simulink model "PathFollowComp"  (R2015a)
settings: Solver=ode3  StartTime=0.0  StopTime=400  FixedStep=0.01  RelTol=1e-3
values from neighbouring files (symbols this model uses):
  K_eta = 1    [CD.m]    (also in PathFollowCompScript.m = 0.21)
  lambda_0 = atan2(lambda_vec_0(2),lambda_vec_0(1))    [CD.m]    (also in PathFollowCompScript.m)
  rangethresh = 50    [PathFollowCompScript.m]
undefined symbols (not defined in the file): Initial_Heading, Initial_Position, Initial_Position_O
libraries: simulink x13, aerolibtransform2 x4
(part 1 of 2)
settings Model: Creator=marinho  LastModifiedBy=marinho

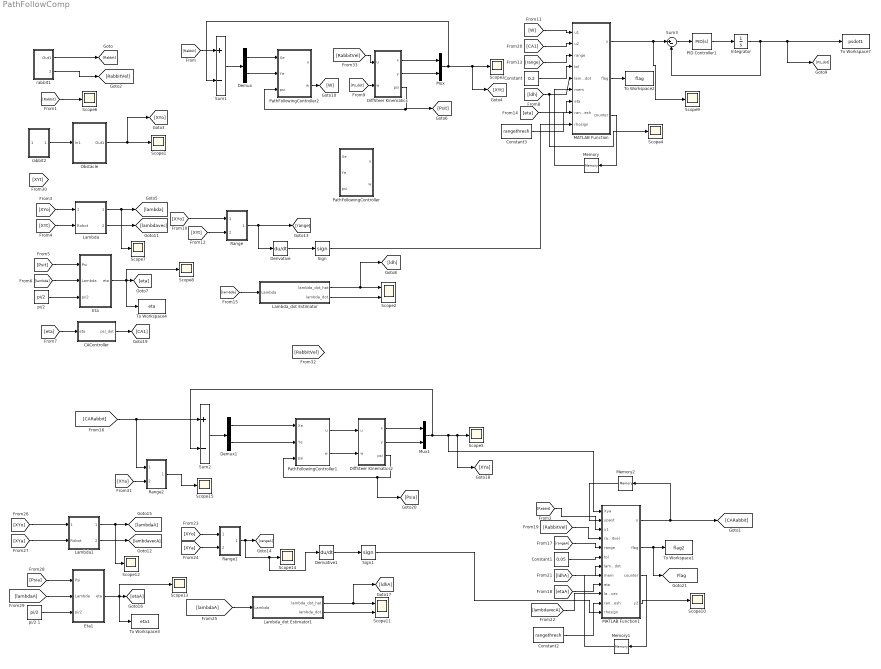
== system PathFollowComp ==
  CAController : Subsystem
  Constant : Constant  Value=0.2
  Constant1 : Constant  Value=0.05
  Constant2 : Constant  Value=rangethresh
  Constant3 : Constant  Value=rangethresh
  Demux : Demux  Outputs=2
  Demux1 : Demux  Outputs=2
  Derivative : Derivative
  Derivative1 : Derivative
  DiffSteer Kinematics : Subsystem  AncestorBlock=DiffSteer_model/DiffSteer Kinematics  mask{x0=[Initial_Position Initial_Heading], a=0.2, umax=32, wmax=5, dumax=inf, dwmax=inf}
      mask prompts: x0 "Initial pose [x, y, psi]"; a "Distance from traction wheels axis center to the point of interest [m]"; umax "Maximum linear velocity [m/s]"; wmax "Maximum angular velocity [rad/s]"; dumax "Maximum linear acceleration [m/s^2]"; dwmax "Maximum angular acceleration [rad/s^2]"
      mask help: Kinematics of the differential steered vehicle
      mask Help:
      | Kinematics of the differential steered vehicle (unicycle-like).
      | 
      | A differential steered (or differential wheeled) robot has two separately driven wheels placed on either side of its structure. Its orientation is changed by varying the relative velocities of its wheels.
      | In this model, robot position [x,y] is the position of the point of interest, which is located on a distance "a" from the center of the line that connects both traction wheels. If a = 0, this model is equal to the unicycle.
      | 
      | <b>Parameters:</b>
      | 
      | Initial pose: Vehicle initial position and orientation on absolute reference frame [x_0, y_0, psi_0]
      | Distance between traction wheels axis and point of interest (1x1): a [m]
      | Maximum Linear velocity (1x1):  Vehicle speed limit [m/s] (umax)
      | Maximum Angular velocity (1x1):  Vehicle turning velocity limit [rad/s] (wmax)
      | Maximum linear acceleration (1x1): Vehicle linear acceleration limit [m/s2] (dumax)
      | Maximum angular acceleration (1x1): Vehicle angular acceleration limit [rad/s2] (dwmax)
      | 
      | 
      | <b>Inputs:</b>
      | 
      | u (1x1): reference for linear velocity [m/s]
      | w (1x1): reference for angular velocity [rad/s]
      | 
      | <b>Outputs:</b>
      | 
      | x (1x1): x-coordinate in world frame [m]
      | y (1x1): y-coordinate in world frame [m]
      | psi (1x1): heading angle in world frame [rad]
      | 
      | <b>Notes:</b>
      | 
      | 1. If a = 0, this model is equal to the unicycle.
      | 
      | 2. This model does not take into account the robot dynamics. It considers that the actual robot velocity is exactly equal to the reference velocity (if it is bellow its limit).
      | 
      | For more information on the robot kinematics and dynamics, please refer to:
      | 
      | [1] MARTINS, F.N., CARELLI, R., SARCINELLI-FILHO, M. and BASTOS-FILHO, T.F.
      | Dynamic Modeling and Adaptive Dynamic Compensation for Unicycle-Like
      | Mobile Robots. 14th International Conference on Advanced Robotics -
      | ICAR 2009, Germany, June, 22-26, 2009.
      | 
      | [2] MARTINS, F.N., CELESTE, W.C., CARELLI, R., SARCINELLI-FILHO, M. and
      | BASTOS-FILHO, T.F. An Adaptive Dynamic Controller for Autonomous Mobile Robot
      | Trajectory Tracking. Control Engineering Practice, v. 16, p. 1354–1363, 2008.
      | doi: 10.1016/j.conengprac.2008.03.004
  DiffSteer Kinematics2 : Subsystem  AncestorBlock=DiffSteer_model/DiffSteer Kinematics  mask{x0=[Initial_Position Initial_Heading], a=0.2, umax=32, wmax=5, dumax=inf, dwmax=inf}
      mask prompts: x0 "Initial pose [x, y, psi]"; a "Distance from traction wheels axis center to the point of interest [m]"; umax "Maximum linear velocity [m/s]"; wmax "Maximum angular velocity [rad/s]"; dumax "Maximum linear acceleration [m/s^2]"; dwmax "Maximum angular acceleration [rad/s^2]"
      mask help: Kinematics of the differential steered vehicle
      mask Help:
      | Kinematics of the differential steered vehicle (unicycle-like).
      | 
      | A differential steered (or differential wheeled) robot has two separately driven wheels placed on either side of its structure. Its orientation is changed by varying the relative velocities of its wheels.
      | In this model, robot position [x,y] is the position of the point of interest, which is located on a distance "a" from the center of the line that connects both traction wheels. If a = 0, this model is equal to the unicycle.
      | 
      | <b>Parameters:</b>
      | 
      | Initial pose: Vehicle initial position and orientation on absolute reference frame [x_0, y_0, psi_0]
      | Distance between traction wheels axis and point of interest (1x1): a [m]
      | Maximum Linear velocity (1x1):  Vehicle speed limit [m/s] (umax)
      | Maximum Angular velocity (1x1):  Vehicle turning velocity limit [rad/s] (wmax)
      | Maximum linear acceleration (1x1): Vehicle linear acceleration limit [m/s2] (dumax)
      | Maximum angular acceleration (1x1): Vehicle angular acceleration limit [rad/s2] (dwmax)
      | 
      | 
      | <b>Inputs:</b>
      | 
      | u (1x1): reference for linear velocity [m/s]
      | w (1x1): reference for angular velocity [rad/s]
      | 
      | <b>Outputs:</b>
      | 
      | x (1x1): x-coordinate in world frame [m]
      | y (1x1): y-coordinate in world frame [m]
      | psi (1x1): heading angle in world frame [rad]
      | 
      | <b>Notes:</b>
      | 
      | 1. If a = 0, this model is equal to the unicycle.
      | 
      | 2. This model does not take into account the robot dynamics. It considers that the actual robot velocity is exactly equal to the reference velocity (if it is bellow its limit).
      | 
      | For more information on the robot kinematics and dynamics, please refer to:
      | 
      | [1] MARTINS, F.N., CARELLI, R., SARCINELLI-FILHO, M. and BASTOS-FILHO, T.F.
      | Dynamic Modeling and Adaptive Dynamic Compensation for Unicycle-Like
      | Mobile Robots. 14th International Conference on Advanced Robotics -
      | ICAR 2009, Germany, June, 22-26, 2009.
      | 
      | [2] MARTINS, F.N., CELESTE, W.C., CARELLI, R., SARCINELLI-FILHO, M. and
      | BASTOS-FILHO, T.F. An Adaptive Dynamic Controller for Autonomous Mobile Robot
      | Trajectory Tracking. Control Engineering Practice, v. 16, p. 1354–1363, 2008.
      | doi: 10.1016/j.conengprac.2008.03.004
  Eta : Subsystem
  Eta1 : Subsystem
  Integrator : Integrator  UpperSaturationLimit=0.5  LowerSaturationLimit=-0.5
  Lambda : Subsystem
  Lambda1 : Subsystem
  Lambda_dot Estimator : Subsystem
  Lambda_dot Estimator1 : Subsystem
  MATLAB Function : MATLAB Function  TreatAsAtomicUnit=on
  MATLAB Function1 : MATLAB Function  TreatAsAtomicUnit=on
  Memory : Memory
  Memory1 : Memory
  Memory2 : Memory  X0=[0 0]'
  Mux : Mux  Inputs=2
  Mux1 : Mux  Inputs=2
  Obstacle : Subsystem
  PID Controller1 : simulink/Continuous/PID Controller  Controller=PID  TimeDomain=Continuous-time  SampleTime=-1  IntegratorMethod=Forward Euler  FilterMethod=Forward Euler  Form=Parallel  UseFilter=on  ControllerParametersSource=internal  P=1  I=0  D=0.05  N=100  InitialConditionSource=internal  InitialConditionForIntegrator=0  InitialConditionForFilter=0  ExternalReset=none  LimitOutput=off  UpperSaturationLimit=0.1  LowerSaturationLimit=-0.1  LinearizeAsGain=on  AntiWindupMode=none  Kb=1  TrackingMode=off  Kt=1  PParamMin=[]  PParamMax=[]  IParamMin=[]  IParamMax=[]  DParamMin=[]  DParamMax=[]  NParamMin=[]  NParamMax=[]  KbParamMin=[]  KbParamMax=[]  KtParamMin=[]  KtParamMax=[]  POutMin=[]  POutMax=[]  IOutMin=[]  IOutMax=[]  DOutMin=[]  DOutMax=[]  NOutMin=[]  NOutMax=[]  KbOutMin=[]  KbOutMax=[]  KtOutMin=[]  KtOutMax=[]  IntegratorOutMin=[]  IntegratorOutMax=[]  FilterOutMin=[]  FilterOutMax=[]  SumOutMin=[]  SumOutMax=[]  SumI1OutMin=[]  SumI1OutMax=[]  SumI2OutMin=[]  SumI2OutMax=[]  SumI3OutMin=[]  SumI3OutMax=[]  SumDOutMin=[]  SumDOutMax=[]  SaturationOutMin=[]  SaturationOutMax=[]  IntegratorContinuousStateAttributes=''  IntegratorStateMustResolveToSignalObject=off  IntegratorRTWStateStorageClass=Auto  FilterContinuousStateAttributes=''  FilterStateMustResolveToSignalObject=off  FilterRTWStateStorageClass=Auto  DifferentiatorICPrevScaledInput=0  DifferentiatorOutMin=[]  DifferentiatorOutMax=[]
  PathFollowingController : Subsystem
  PathFollowingController1 : Subsystem
  PathFollowingController2 : Subsystem
  Range : Subsystem
  Range1 : Subsystem
  Range2 : Subsystem
  Scope{1,3..10,12..15} (13 alike) : Scope
      Scope1 settings: YMin=-250  YMax=25  SaveName=Obstacle
      Scope10 settings: SaveName=NewRabbit
      Scope12 settings: SaveName=Cdc5  DataFormat=Structure
      Scope13 settings: SaveName=Cdc6  DataFormat=Structure
      Scope14 settings: YMin=50  YMax=425  SaveName=Range
      Scope15 settings: YMin=85  YMax=160  SaveName=NewRabbit1
      Scope3 settings: SaveName=Cdc  DataFormat=Structure
      Scope4 settings: SaveName=Cdc1  DataFormat=Structure
      Scope5 settings: SaveName=AlphaBased  DataFormat=Structure
      Scope6 settings: SaveName=Rabbit
      Scope7 settings: SaveName=Cdc2  DataFormat=Structure
      Scope8 settings: SaveName=Cdc3  DataFormat=Structure
      Scope9 settings: SaveName=Cdc4  DataFormat=Structure
  Scope11 : Scope  NumInputPorts=2
      settings: YMin=-5~-5  YMax=5~5
  Scope2 : Scope  NumInputPorts=2
      settings: YMin=-1~-5  YMax=12~70  SaveName=ScopeData10
  Sign : Signum
  Sign1 : Signum
  Sum1 : Sum  Inputs=+-
  Sum2 : Sum  Inputs=+-
  Sum3 : Sum  Inputs=|+-
  To Workspace1 : ToWorkspace  VariableName=flag2  SampleTime=-1
  To Workspace2 : ToWorkspace  VariableName=flag  SampleTime=-1
  To Workspace3 : ToWorkspace  VariableName=eta1  SampleTime=-1
  To Workspace4 : ToWorkspace  VariableName=eta  SampleTime=-1
  To Workspace7 : ToWorkspace  VariableName=psdot1  SampleTime=-1
  "pi/2 " : Constant  Value=pi/2  VectorParams1D=off  SampleTime=-1
  pi/2 1 : Constant  Value=pi/2  VectorParams1D=off  SampleTime=-1
  rabbit1 : Subsystem
  rabbit2 : Subsystem
  tag scope: Flag=global
  wires:
  DiffSteer Kinematics/1(x) -> Mux/1
  DiffSteer Kinematics/2(y) -> Mux/2
  Sum1/1 -> Demux/1
  Demux/2 -> PathFollowingController2/2(Ye)
  Demux/1 -> PathFollowingController2/1(Xe)
  Mux/1 -> Sum1/2, [XYt], Scope3/1
  DiffSteer Kinematics/3(psi) -> PathFollowingController2/3(psi), [Psit]
  DiffSteer Kinematics2/1(x) -> Mux1/1
  DiffSteer Kinematics2/2(y) -> Mux1/2
  Sum2/1 -> Demux1/1
  Demux1/2 -> PathFollowingController1/2(Ye)
  Demux1/1 -> PathFollowingController1/1(Xe)
  Mux1/1 -> Sum2/2, MATLAB Function1/1(Xya), [XYa], Scope5/1
  PathFollowingController1/2(w) -> DiffSteer Kinematics2/2(w)
  DiffSteer Kinematics2/3(psi) -> [Psia], PathFollowingController1/3(psi)
  rabbit1/1(Out1) -> [Rabbit]
  [Rabbit] -> Sum1/1
  [Rabbit] -> Scope6/1
  [XYo] -> Lambda/1(Object)
  [XYt] -> Lambda/2(Robot)
  Lambda/1(Lambda) -> Scope7/1, [lambda]
  Eta/1(eta) -> To Workspace4/1, Scope8/1, [eta]
  [Psit] -> Eta/1(Psi)
  [lambda] -> Eta/2(Lambda)
  "pi/2 "/1 -> Eta/3(pi/2)
  [eta] -> CAController/1(eta)
  CAController/1(psi_dot) -> [CA1]
  [W] -> MATLAB Function/1(u1)
  MATLAB Function/2(flag) -> To Workspace2/1
  [range] -> MATLAB Function/3(range)
  MATLAB Function/3(counter) -> Memory/1
  Memory/1 -> MATLAB Function/6(mem)
  Constant/1 -> MATLAB Function/4(tol)
  [eta] -> MATLAB Function/7(eta)
  [ldh] -> Scope4/1, MATLAB Function/5(lambda_dot)
  Sum3/1 -> PID Controller1/1
  PID Controller1/1 -> Integrator/1
  MATLAB Function/1(y) -> Scope9/1, Sum3/1
  Integrator/1 -> [Ps_dot], To Workspace7/1, Sum3/2
  [CA1] -> MATLAB Function/2(u2)
  PathFollowingController2/2(w) -> [W]
  [Ps_dot] -> DiffSteer Kinematics/2(w)
  [XYo] -> Range/1(In1)
  [XYt] -> Range/2(In2)
  Range/1(Out1) -> Derivative/1, [range]
  [lambda] -> Lambda_dot Estimator/1(Lambda)
  Lambda_dot Estimator/1(lambda_dot_hat) -> [ldh], Scope2/1
  Lambda_dot Estimator/2(lambda_dot) -> Scope2/2
  [Rabbit] -> MATLAB Function1/3(u1)
  [rangeA] -> MATLAB Function1/5(range)
  MATLAB Function1/3(counter) -> Memory1/1
  Memory1/1 -> MATLAB Function1/8(mem)
  Constant1/1 -> MATLAB Function1/6(tol)
  [etaA] -> MATLAB Function1/9(eta)
  [ldhA] -> MATLAB Function1/7(lambda_dot)
  MATLAB Function1/1(y) -> Memory2/1, [CARabbit]
  [CARabbit] -> Range2/1(In1), Sum2/1
  rabbit1/2(Velocity) -> [RabbitVel]
  [RabbitVel] -> MATLAB Function1/4(rabbitvel)
  Lambda/2(LambdaVec) -> [lambdavec]
  [lambdavecA] -> MATLAB Function1/10(lambdavec)
  MATLAB Function1/4(y2) -> Scope10/1
  Memory2/1 -> MATLAB Function1/2(ypast)
  Constant2/1 -> MATLAB Function1/11(rangethresh)
  Constant3/1 -> MATLAB Function/8(rangethresh)
  [XYo] -> Lambda1/1(Object)
  [XYa] -> Lambda1/2(Robot)
  Lambda1/1(Lambda) -> Scope12/1, [lambdaA]
  Eta1/1(eta) -> To Workspace3/1, Scope13/1, [etaA]
  [Psia] -> Eta1/1(Psi)
  [lambdaA] -> Eta1/2(Lambda)
  pi/2 1/1 -> Eta1/3(pi/2)
  [XYo] -> Range1/1(In1)
  [XYa] -> Range1/2(In2)
  Range1/1(Out1) -> Derivative1/1, Scope14/1, [rangeA]
  [lambdaA] -> Lambda_dot Estimator1/1(Lambda)
  Lambda_dot Estimator1/1(lambda_dot_hat) -> [ldhA], Scope11/1
  Lambda_dot Estimator1/2(lambda_dot) -> Scope11/2
  Lambda1/2(LambdaVec) -> [lambdavecA]
  Obstacle/1(Out1) -> [XYo], Scope1/1
  Derivative/1 -> Sign/1
  Sign/1 -> MATLAB Function/9(rhosign)
  Derivative1/1 -> Sign1/1
  Sign1/1 -> MATLAB Function1/12(rhosign)
  [XYa] -> Range2/2(In2)
  Range2/1(Out1) -> Scope15/1
  MATLAB Function1/2(flag) -> [Flag], To Workspace1/1
  rabbit2/1(Out1) -> Obstacle/1(In1)
  [RabbitVel] -> DiffSteer Kinematics/1(u)
  PathFollowingController1/1(u) -> DiffSteer Kinematics2/1(u)

== system PathFollowComp/CAController ==
  eta : Inport
  Gain : Gain  Gain=-K_eta
  psi_dot : Outport
  wires:
  Gain/1 -> psi_dot/1
  eta/1 -> Gain/1

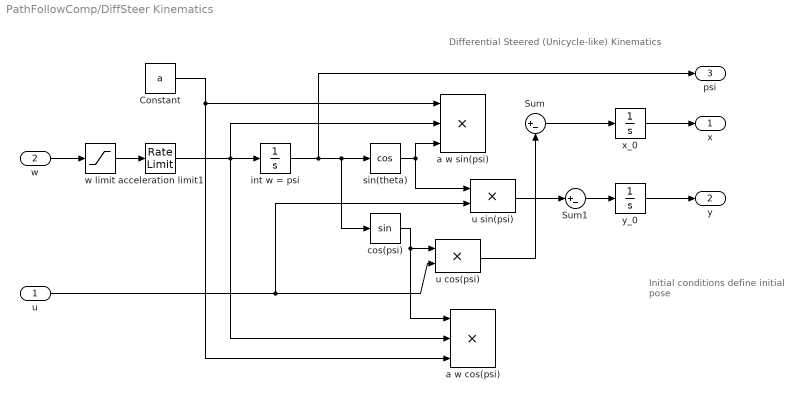
== system PathFollowComp/DiffSteer Kinematics ==
  note: Initial conditions define
      | initial pose
  note: Differential Steered (Unicycle-like) Kinematics
  u : Inport
  w : Inport  Port=2
  Constant : Constant  Value=a
  Sum : Sum  Inputs=|+-  SaturateOnIntegerOverflow=on
  Sum1 : Sum  Inputs=|+-  SaturateOnIntegerOverflow=on
  a w cos(psi) : Product  Inputs=3  SaturateOnIntegerOverflow=on  OutDataTypeStr=Inherit: Same as first input
  a w sin(psi) : Product  Inputs=3  SaturateOnIntegerOverflow=on  OutDataTypeStr=Inherit: Same as first input
  acceleration limit1 : RateLimiter  RisingSlewLimit=dwmax  FallingSlewLimit=-dwmax  SampleTimeMode=inherited
  cos(psi) : Trigonometry
  int w = psi : Integrator  InitialCondition=x0(3)
  sin(theta) : Trigonometry  Operator=cos
  u cos(psi) : Product  SaturateOnIntegerOverflow=on  OutDataTypeStr=Inherit: Same as first input
  u sin(psi) : Product  SaturateOnIntegerOverflow=on  OutDataTypeStr=Inherit: Same as first input
  w limit : Saturate  UpperLimit=wmax  LowerLimit=-wmax
  x_0 : Integrator  InitialCondition=x0(1)
  y_0 : Integrator  InitialCondition=x0(2)
  x : Outport
  y : Outport  Port=2
  psi : Outport  Port=3
  wires:
  w limit/1 -> acceleration limit1/1
  w/1 -> w limit/1
  u cos(psi)/1 -> Sum/2
  u sin(psi)/1 -> Sum1/1
  cos(psi)/1 -> u cos(psi)/1, a w cos(psi)/1
  acceleration limit1/1 -> a w sin(psi)/2, int w = psi/1, a w cos(psi)/2
  Constant/1 -> a w sin(psi)/1, a w cos(psi)/3
  x_0/1 -> x/1
  Sum/1 -> x_0/1
  sin(theta)/1 -> a w sin(psi)/3, u sin(psi)/1
  int w = psi/1 -> psi/1, sin(theta)/1, cos(psi)/1
  u/1 -> u sin(psi)/2, u cos(psi)/2
  Sum1/1 -> y_0/1
  y_0/1 -> y/1

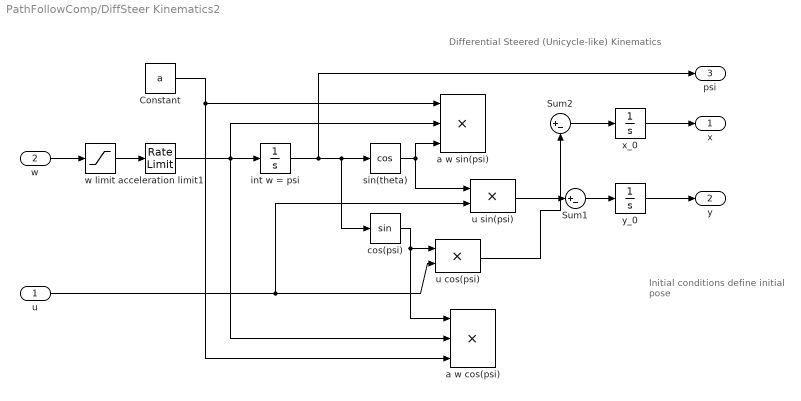
== system PathFollowComp/DiffSteer Kinematics2 ==
  note: Initial conditions define
      | initial pose
  note: Differential Steered (Unicycle-like) Kinematics
  u : Inport
  w : Inport  Port=2
  Constant : Constant  Value=a
  Sum1 : Sum  Inputs=|+-  SaturateOnIntegerOverflow=on
  Sum2 : Sum  Inputs=|+-  SaturateOnIntegerOverflow=on
  a w cos(psi) : Product  Inputs=3  SaturateOnIntegerOverflow=on  OutDataTypeStr=Inherit: Same as first input
  a w sin(psi) : Product  Inputs=3  SaturateOnIntegerOverflow=on  OutDataTypeStr=Inherit: Same as first input
  acceleration limit1 : RateLimiter  RisingSlewLimit=dwmax  FallingSlewLimit=-dwmax  SampleTimeMode=inherited
  cos(psi) : Trigonometry
  int w = psi : Integrator  InitialCondition=x0(3)
  sin(theta) : Trigonometry  Operator=cos
  u cos(psi) : Product  SaturateOnIntegerOverflow=on  OutDataTypeStr=Inherit: Same as first input
  u sin(psi) : Product  SaturateOnIntegerOverflow=on  OutDataTypeStr=Inherit: Same as first input
  w limit : Saturate  UpperLimit=wmax  LowerLimit=-wmax
  x_0 : Integrator  InitialCondition=x0(1)
  y_0 : Integrator  InitialCondition=x0(2)
  x : Outport
  y : Outport  Port=2
  psi : Outport  Port=3
  wires:
  w limit/1 -> acceleration limit1/1
  w/1 -> w limit/1
  u sin(psi)/1 -> Sum1/1
  cos(psi)/1 -> u cos(psi)/1, a w cos(psi)/1
  acceleration limit1/1 -> a w sin(psi)/2, int w = psi/1, a w cos(psi)/2
  Constant/1 -> a w sin(psi)/1, a w cos(psi)/3
  x_0/1 -> x/1
  u cos(psi)/1 -> Sum2/2
  sin(theta)/1 -> a w sin(psi)/3, u sin(psi)/1
  int w = psi/1 -> psi/1, sin(theta)/1, cos(psi)/1
  u/1 -> u sin(psi)/2, u cos(psi)/2
  Sum1/1 -> y_0/1
  y_0/1 -> y/1
  Sum2/1 -> x_0/1

== system PathFollowComp/Eta ==
  Psi : Inport
  Lambda : Inport  Port=2
  pi/2 : Inport  Port=3
  Gain5 : Gain
  Sum2 : Sum  Inputs=+-
  Sum3 : Sum  Inputs=+-
  wrap1 : MATLAB Function  TreatAsAtomicUnit=on
  eta : Outport
  wires:
  wrap1/1(y) -> eta/1
  Psi/1 -> Gain5/1
  Lambda/1 -> Sum3/1
  Sum3/1 -> Sum2/2
  pi/2/1 -> Sum3/2
  Sum2/1 -> wrap1/1(u)
  Gain5/1 -> Sum2/1

== system PathFollowComp/Eta1 ==
  Psi : Inport
  Lambda : Inport  Port=2
  pi/2 : Inport  Port=3
  Gain5 : Gain
  Sum2 : Sum  Inputs=+-
  Sum3 : Sum  Inputs=+-
  wrap1 : MATLAB Function  TreatAsAtomicUnit=on
  eta : Outport
  wires:
  wrap1/1(y) -> eta/1
  Psi/1 -> Gain5/1
  Lambda/1 -> Sum3/1
  Sum3/1 -> Sum2/2
  pi/2/1 -> Sum3/2
  Sum2/1 -> wrap1/1(u)
  Gain5/1 -> Sum2/1

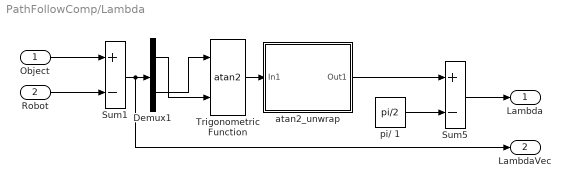
== system PathFollowComp/Lambda ==
  Object : Inport
  Robot : Inport  Port=2
  Demux1 : Demux  Outputs=2
  Sum1 : Sum  Inputs=+-
  Sum5 : Sum  Inputs=+-
  Trigonometric Function : Trigonometry  Operator=atan2
  atan2_unwrap : Subsystem
  pi/ 1 : Constant  Value=pi/2  VectorParams1D=off  SampleTime=-1
  Lambda : Outport
  LambdaVec : Outport  Port=2
  wires:
  Trigonometric Function/1 -> atan2_unwrap/1(In1)
  Demux1/2 -> Trigonometric Function/1
  pi/ 1/1 -> Sum5/2
  Sum5/1 -> Lambda/1
  atan2_unwrap/1(Out1) -> Sum5/1
  Sum1/1 -> LambdaVec/1, Demux1/1
  Demux1/1 -> Trigonometric Function/2
  Object/1 -> Sum1/1
  Robot/1 -> Sum1/2

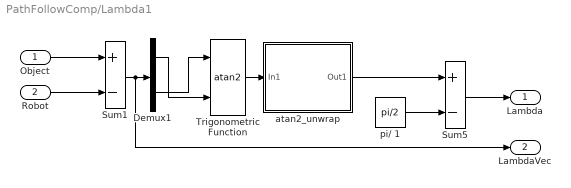
== system PathFollowComp/Lambda1 ==
  Object : Inport
  Robot : Inport  Port=2
  Demux1 : Demux  Outputs=2
  Sum1 : Sum  Inputs=+-
  Sum5 : Sum  Inputs=+-
  Trigonometric Function : Trigonometry  Operator=atan2
  atan2_unwrap : Subsystem
  pi/ 1 : Constant  Value=pi/2  VectorParams1D=off  SampleTime=-1
  Lambda : Outport
  LambdaVec : Outport  Port=2
  wires:
  Trigonometric Function/1 -> atan2_unwrap/1(In1)
  Demux1/2 -> Trigonometric Function/1
  pi/ 1/1 -> Sum5/2
  Sum5/1 -> Lambda/1
  atan2_unwrap/1(Out1) -> Sum5/1
  Sum1/1 -> LambdaVec/1, Demux1/1
  Demux1/1 -> Trigonometric Function/2
  Object/1 -> Sum1/1
  Robot/1 -> Sum1/2

== system PathFollowComp/Lambda_dot Estimator ==
  Lambda : Inport
  Derivative : Derivative
  Gain2 : Gain  Gain=5
  Integrator : Integrator
  Scope : Scope
  Sum5 : Sum  Inputs=|+-
  lambda_dot_hat : Outport
  lambda_dot : Outport  Port=2
  wires:
  Sum5/1 -> Scope/1, Gain2/1
  Gain2/1 -> lambda_dot_hat/1, Integrator/1
  Integrator/1 -> Sum5/2
  Lambda/1 -> Derivative/1, Sum5/1
  Derivative/1 -> lambda_dot/1

== system PathFollowComp/Lambda_dot Estimator1 ==
  Lambda : Inport
  Derivative : Derivative
  Gain2 : Gain  Gain=5
  Integrator : Integrator
  Scope : Scope
  Sum5 : Sum  Inputs=|+-
  lambda_dot_hat : Outport
  lambda_dot : Outport  Port=2
  wires:
  Sum5/1 -> Scope/1, Gain2/1
  Gain2/1 -> lambda_dot_hat/1, Integrator/1
  Integrator/1 -> Sum5/2
  Lambda/1 -> Derivative/1, Sum5/1
  Derivative/1 -> lambda_dot/1

== system PathFollowComp/Obstacle ==
  In1 : Inport
  Demux2 : Demux  Outputs=2
  DiffSteer Kinematics1 : Subsystem  AncestorBlock=DiffSteer_model/DiffSteer Kinematics  mask{x0=[Initial_Position_O Initial_Heading], a=0.2, umax=6, wmax=5, dumax=inf, dwmax=inf}
      mask prompts: x0 "Initial pose [x, y, psi]"; a "Distance from traction wheels axis center to the point of interest [m]"; umax "Maximum linear velocity [m/s]"; wmax "Maximum angular velocity [rad/s]"; dumax "Maximum linear acceleration [m/s^2]"; dwmax "Maximum angular acceleration [rad/s^2]"
      mask help: Kinematics of the differential steered vehicle
      mask Help:
      | Kinematics of the differential steered vehicle (unicycle-like).
      | 
      | A differential steered (or differential wheeled) robot has two separately driven wheels placed on either side of its structure. Its orientation is changed by varying the relative velocities of its wheels.
      | In this model, robot position [x,y] is the position of the point of interest, which is located on a distance "a" from the center of the line that connects both traction wheels. If a = 0, this model is equal to the unicycle.
      | 
      | <b>Parameters:</b>
      | 
      | Initial pose: Vehicle initial position and orientation on absolute reference frame [x_0, y_0, psi_0]
      | Distance between traction wheels axis and point of interest (1x1): a [m]
      | Maximum Linear velocity (1x1):  Vehicle speed limit [m/s] (umax)
      | Maximum Angular velocity (1x1):  Vehicle turning velocity limit [rad/s] (wmax)
      | Maximum linear acceleration (1x1): Vehicle linear acceleration limit [m/s2] (dumax)
      | Maximum angular acceleration (1x1): Vehicle angular acceleration limit [rad/s2] (dwmax)
      | 
      | 
      | <b>Inputs:</b>
      | 
      | u (1x1): reference for linear velocity [m/s]
      | w (1x1): reference for angular velocity [rad/s]
      | 
      | <b>Outputs:</b>
      | 
      | x (1x1): x-coordinate in world frame [m]
      | y (1x1): y-coordinate in world frame [m]
      | psi (1x1): heading angle in world frame [rad]
      | 
      | <b>Notes:</b>
      | 
      | 1. If a = 0, this model is equal to the unicycle.
      | 
      | 2. This model does not take into account the robot dynamics. It considers that the actual robot velocity is exactly equal to the reference velocity (if it is bellow its limit).
      | 
      | For more information on the robot kinematics and dynamics, please refer to:
      | 
      | [1] MARTINS, F.N., CARELLI, R., SARCINELLI-FILHO, M. and BASTOS-FILHO, T.F.
      | Dynamic Modeling and Adaptive Dynamic Compensation for Unicycle-Like
      | Mobile Robots. 14th International Conference on Advanced Robotics -
      | ICAR 2009, Germany, June, 22-26, 2009.
      | 
      | [2] MARTINS, F.N., CELESTE, W.C., CARELLI, R., SARCINELLI-FILHO, M. and
      | BASTOS-FILHO, T.F. An Adaptive Dynamic Controller for Autonomous Mobile Robot
      | Trajectory Tracking. Control Engineering Practice, v. 16, p. 1354–1363, 2008.
      | doi: 10.1016/j.conengprac.2008.03.004
  Mux2 : Mux  Inputs=2
  PathFollowingController2 : Subsystem
  Scope : Scope
      settings: SaveName=ScopeData2
  Sum3 : Sum  Inputs=+-
  Out1 : Outport
  wires:
  DiffSteer Kinematics1/1(x) -> Mux2/1
  DiffSteer Kinematics1/2(y) -> Mux2/2
  Sum3/1 -> Demux2/1
  Demux2/2 -> PathFollowingController2/2(Ye)
  Demux2/1 -> PathFollowingController2/1(Xe)
  Mux2/1 -> Out1/1, Sum3/2
  PathFollowingController2/2(w) -> DiffSteer Kinematics1/2(w)
  DiffSteer Kinematics1/3(psi) -> PathFollowingController2/3(psi)
  PathFollowingController2/1(u) -> Scope/1, DiffSteer Kinematics1/1(u)
  In1/1 -> Sum3/1

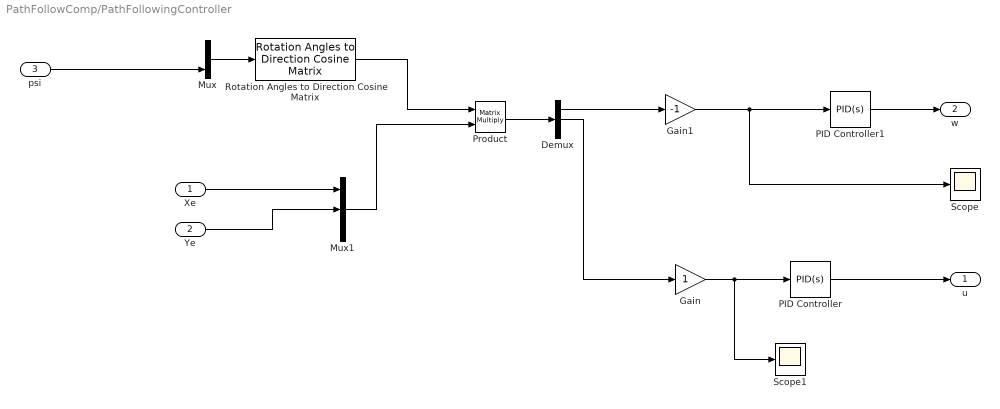
== system PathFollowComp/PathFollowingController ==
  Xe : Inport
  Ye : Inport  Port=2
  psi : Inport  Port=3
  Demux : Demux  Outputs=3
  Gain : Gain
  Gain1 : Gain  Gain=-1
  Mux : Mux  Inputs=3
  Mux1 : Mux  Inputs=3
  PID Controller : simulink/Continuous/PID Controller  Controller=PID  TimeDomain=Continuous-time  SampleTime=-1  IntegratorMethod=Forward Euler  FilterMethod=Forward Euler  Form=Parallel  UseFilter=on  ControllerParametersSource=internal  P=0.1  I=0.0001  D=0  N=100  InitialConditionSource=internal  InitialConditionForIntegrator=0  InitialConditionForFilter=0  ExternalReset=none  LimitOutput=on  UpperSaturationLimit=10  LowerSaturationLimit=0  LinearizeAsGain=on  AntiWindupMode=none  Kb=1  TrackingMode=off  Kt=1  PParamMin=[]  PParamMax=[]  IParamMin=[]  IParamMax=[]  DParamMin=[]  DParamMax=[]  NParamMin=[]  NParamMax=[]  KbParamMin=[]  KbParamMax=[]  KtParamMin=[]  KtParamMax=[]  POutMin=[]  POutMax=[]  IOutMin=[]  IOutMax=[]  DOutMin=[]  DOutMax=[]  NOutMin=[]  NOutMax=[]  KbOutMin=[]  KbOutMax=[]  KtOutMin=[]  KtOutMax=[]  IntegratorOutMin=[]  IntegratorOutMax=[]  FilterOutMin=[]  FilterOutMax=[]  SumOutMin=[]  SumOutMax=[]  SumI1OutMin=[]  SumI1OutMax=[]  SumI2OutMin=[]  SumI2OutMax=[]  SumI3OutMin=[]  SumI3OutMax=[]  SumDOutMin=[]  SumDOutMax=[]  SaturationOutMin=[]  SaturationOutMax=[]  IntegratorContinuousStateAttributes=''  IntegratorStateMustResolveToSignalObject=off  IntegratorRTWStateStorageClass=Auto  FilterContinuousStateAttributes=''  FilterStateMustResolveToSignalObject=off  FilterRTWStateStorageClass=Auto  DifferentiatorICPrevScaledInput=0  DifferentiatorOutMin=[]  DifferentiatorOutMax=[]
  PID Controller1 : simulink/Continuous/PID Controller  Controller=PID  TimeDomain=Continuous-time  SampleTime=-1  IntegratorMethod=Forward Euler  FilterMethod=Forward Euler  Form=Parallel  UseFilter=on  ControllerParametersSource=internal  P=0.04  I=0.0001  D=0.03  N=100  InitialConditionSource=internal  InitialConditionForIntegrator=0  InitialConditionForFilter=0  ExternalReset=none  LimitOutput=on  UpperSaturationLimit=0.2  LowerSaturationLimit=-0.2  LinearizeAsGain=on  AntiWindupMode=none  Kb=1  TrackingMode=off  Kt=1  PParamMin=[]  PParamMax=[]  IParamMin=[]  IParamMax=[]  DParamMin=[]  DParamMax=[]  NParamMin=[]  NParamMax=[]  KbParamMin=[]  KbParamMax=[]  KtParamMin=[]  KtParamMax=[]  POutMin=[]  POutMax=[]  IOutMin=[]  IOutMax=[]  DOutMin=[]  DOutMax=[]  NOutMin=[]  NOutMax=[]  KbOutMin=[]  KbOutMax=[]  KtOutMin=[]  KtOutMax=[]  IntegratorOutMin=[]  IntegratorOutMax=[]  FilterOutMin=[]  FilterOutMax=[]  SumOutMin=[]  SumOutMax=[]  SumI1OutMin=[]  SumI1OutMax=[]  SumI2OutMin=[]  SumI2OutMax=[]  SumI3OutMin=[]  SumI3OutMax=[]  SumDOutMin=[]  SumDOutMax=[]  SaturationOutMin=[]  SaturationOutMax=[]  IntegratorContinuousStateAttributes=''  IntegratorStateMustResolveToSignalObject=off  IntegratorRTWStateStorageClass=Auto  FilterContinuousStateAttributes=''  FilterStateMustResolveToSignalObject=off  FilterRTWStateStorageClass=Auto  DifferentiatorICPrevScaledInput=0  DifferentiatorOutMin=[]  DifferentiatorOutMax=[]
  Product : Product  Multiplication=Matrix(*)
  Rotation Angles to Direction Cosine Matrix : aerolibtransform2/Rotation Angles to Direction Cosine Matrix  rotationOrder=XYZ
  Scope : Scope
      settings: SaveName=ScopeData5
  Scope1 : Scope
      settings: YMin=8750  YMax=12500  SaveName=ScopeData6
  u : Outport
  w : Outport  Port=2
  wires:
  PID Controller/1 -> u/1
  Ye/1 -> Mux1/2
  Xe/1 -> Mux1/1
  PID Controller1/1 -> w/1
  Gain1/1 -> PID Controller1/1, Scope/1
  Gain/1 -> PID Controller/1, Scope1/1
  Demux/2 -> Gain/1
  Demux/1 -> Gain1/1
  Product/1 -> Demux/1
  Mux1/1 -> Product/2
  Rotation Angles to Direction Cosine Matrix/1 -> Product/1
  Mux/1 -> Rotation Angles to Direction Cosine Matrix/1
  psi/1 -> Mux/3

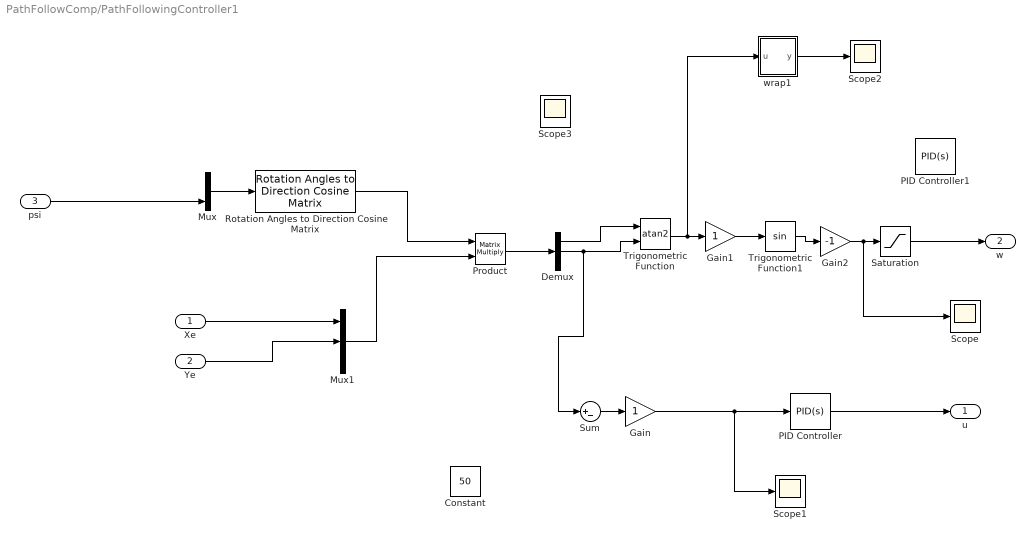
== system PathFollowComp/PathFollowingController1 ==
  Xe : Inport
  Ye : Inport  Port=2
  psi : Inport  Port=3
  Constant : Constant  Value=50
  Demux : Demux  Outputs=3
  Gain : Gain
  Gain1 : Gain
  Gain2 : Gain  Gain=-1
  Mux : Mux  Inputs=3
  Mux1 : Mux  Inputs=3
  PID Controller : simulink/Continuous/PID Controller  Controller=PID  TimeDomain=Continuous-time  SampleTime=-1  IntegratorMethod=Forward Euler  FilterMethod=Forward Euler  Form=Parallel  UseFilter=on  ControllerParametersSource=internal  P=0.1  I=0  D=0  N=100  InitialConditionSource=internal  InitialConditionForIntegrator=0  InitialConditionForFilter=0  ExternalReset=none  LimitOutput=on  UpperSaturationLimit=8  LowerSaturationLimit=0  LinearizeAsGain=on  AntiWindupMode=none  Kb=1  TrackingMode=off  Kt=1  PParamMin=[]  PParamMax=[]  IParamMin=[]  IParamMax=[]  DParamMin=[]  DParamMax=[]  NParamMin=[]  NParamMax=[]  KbParamMin=[]  KbParamMax=[]  KtParamMin=[]  KtParamMax=[]  POutMin=[]  POutMax=[]  IOutMin=[]  IOutMax=[]  DOutMin=[]  DOutMax=[]  NOutMin=[]  NOutMax=[]  KbOutMin=[]  KbOutMax=[]  KtOutMin=[]  KtOutMax=[]  IntegratorOutMin=[]  IntegratorOutMax=[]  FilterOutMin=[]  FilterOutMax=[]  SumOutMin=[]  SumOutMax=[]  SumI1OutMin=[]  SumI1OutMax=[]  SumI2OutMin=[]  SumI2OutMax=[]  SumI3OutMin=[]  SumI3OutMax=[]  SumDOutMin=[]  SumDOutMax=[]  SaturationOutMin=[]  SaturationOutMax=[]  IntegratorContinuousStateAttributes=''  IntegratorStateMustResolveToSignalObject=off  IntegratorRTWStateStorageClass=Auto  FilterContinuousStateAttributes=''  FilterStateMustResolveToSignalObject=off  FilterRTWStateStorageClass=Auto  DifferentiatorICPrevScaledInput=0  DifferentiatorOutMin=[]  DifferentiatorOutMax=[]
  PID Controller1 : simulink/Continuous/PID Controller  Controller=PID  TimeDomain=Continuous-time  SampleTime=-1  IntegratorMethod=Forward Euler  FilterMethod=Forward Euler  Form=Parallel  UseFilter=on  ControllerParametersSource=internal  P=0.1  I=0  D=0  N=100  InitialConditionSource=internal  InitialConditionForIntegrator=0  InitialConditionForFilter=0  ExternalReset=none  LimitOutput=on  UpperSaturationLimit=0.2  LowerSaturationLimit=-0.2  LinearizeAsGain=on  AntiWindupMode=none  Kb=1  TrackingMode=off  Kt=1  PParamMin=[]  PParamMax=[]  IParamMin=[]  IParamMax=[]  DParamMin=[]  DParamMax=[]  NParamMin=[]  NParamMax=[]  KbParamMin=[]  KbParamMax=[]  KtParamMin=[]  KtParamMax=[]  POutMin=[]  POutMax=[]  IOutMin=[]  IOutMax=[]  DOutMin=[]  DOutMax=[]  NOutMin=[]  NOutMax=[]  KbOutMin=[]  KbOutMax=[]  KtOutMin=[]  KtOutMax=[]  IntegratorOutMin=[]  IntegratorOutMax=[]  FilterOutMin=[]  FilterOutMax=[]  SumOutMin=[]  SumOutMax=[]  SumI1OutMin=[]  SumI1OutMax=[]  SumI2OutMin=[]  SumI2OutMax=[]  SumI3OutMin=[]  SumI3OutMax=[]  SumDOutMin=[]  SumDOutMax=[]  SaturationOutMin=[]  SaturationOutMax=[]  IntegratorContinuousStateAttributes=''  IntegratorStateMustResolveToSignalObject=off  IntegratorRTWStateStorageClass=Auto  FilterContinuousStateAttributes=''  FilterStateMustResolveToSignalObject=off  FilterRTWStateStorageClass=Auto  DifferentiatorICPrevScaledInput=0  DifferentiatorOutMin=[]  DifferentiatorOutMax=[]
  Product : Product  Multiplication=Matrix(*)
  Rotation Angles to Direction Cosine Matrix : aerolibtransform2/Rotation Angles to Direction Cosine Matrix  rotationOrder=XYZ
  Saturation : Saturate  UpperLimit=0.4  LowerLimit=-0.4
  Scope{,1..3} (4 alike) : Scope
      Scope settings: SaveName=ScopeData5
      Scope1 settings: YMin=-125  YMax=200  SaveName=ScopeData6
      Scope2 settings: YMin=5.55112e-17  YMax=1.5  SaveName=ScopeData8
      Scope3 settings: YMin=-35  YMax=40  SaveName=ScopeData9
  Sum : Sum  Inputs=|+-
  Trigonometric Function : Trigonometry  Operator=atan2
  Trigonometric Function1 : Trigonometry
  wrap1 : MATLAB Function  TreatAsAtomicUnit=on
  u : Outport
  w : Outport  Port=2
  wires:
  PID Controller/1 -> u/1
  Ye/1 -> Mux1/2
  Xe/1 -> Mux1/1
  Gain2/1 -> Saturation/1, Scope/1
  Gain1/1 -> Trigonometric Function1/1
  Gain/1 -> PID Controller/1, Scope1/1
  Demux/2 -> Sum/1, Trigonometric Function/2
  Product/1 -> Demux/1
  Mux1/1 -> Product/2
  Rotation Angles to Direction Cosine Matrix/1 -> Product/1
  Mux/1 -> Rotation Angles to Direction Cosine Matrix/1
  psi/1 -> Mux/3
  Trigonometric Function/1 -> wrap1/1(u), Gain1/1
  Trigonometric Function1/1 -> Gain2/1
  wrap1/1(y) -> Scope2/1
  Demux/1 -> Trigonometric Function/1
  Saturation/1 -> w/1
  Sum/1 -> Gain/1

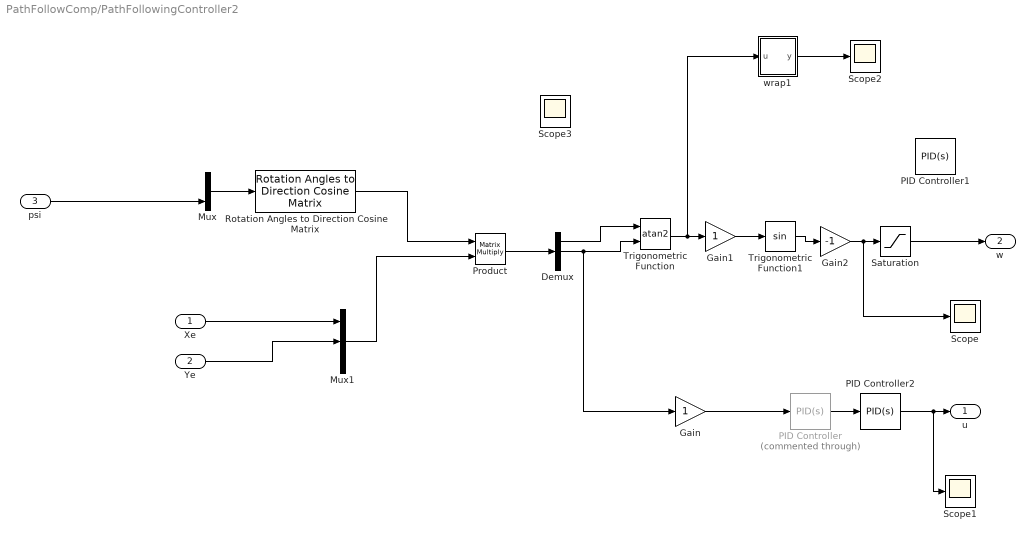
== system PathFollowComp/PathFollowingController2 ==
  Xe : Inport
  Ye : Inport  Port=2
  psi : Inport  Port=3
  Demux : Demux  Outputs=3
  Gain : Gain
  Gain1 : Gain
  Gain2 : Gain  Gain=-1
  Mux : Mux  Inputs=3
  Mux1 : Mux  Inputs=3
  PID Controller : simulink/Continuous/PID Controller  Commented=through  Controller=PID  TimeDomain=Continuous-time  SampleTime=-1  IntegratorMethod=Forward Euler  FilterMethod=Forward Euler  Form=Parallel  UseFilter=on  ControllerParametersSource=internal  P=0.1  I=0  D=0  N=100  InitialConditionSource=internal  InitialConditionForIntegrator=0  InitialConditionForFilter=0  ExternalReset=none  LimitOutput=on  UpperSaturationLimit=5  LowerSaturationLimit=0  LinearizeAsGain=on  AntiWindupMode=none  Kb=1  TrackingMode=off  Kt=1  PParamMin=[]  PParamMax=[]  IParamMin=[]  IParamMax=[]  DParamMin=[]  DParamMax=[]  NParamMin=[]  NParamMax=[]  KbParamMin=[]  KbParamMax=[]  KtParamMin=[]  KtParamMax=[]  POutMin=[]  POutMax=[]  IOutMin=[]  IOutMax=[]  DOutMin=[]  DOutMax=[]  NOutMin=[]  NOutMax=[]  KbOutMin=[]  KbOutMax=[]  KtOutMin=[]  KtOutMax=[]  IntegratorOutMin=[]  IntegratorOutMax=[]  FilterOutMin=[]  FilterOutMax=[]  SumOutMin=[]  SumOutMax=[]  SumI1OutMin=[]  SumI1OutMax=[]  SumI2OutMin=[]  SumI2OutMax=[]  SumI3OutMin=[]  SumI3OutMax=[]  SumDOutMin=[]  SumDOutMax=[]  SaturationOutMin=[]  SaturationOutMax=[]  IntegratorContinuousStateAttributes=''  IntegratorStateMustResolveToSignalObject=off  IntegratorRTWStateStorageClass=Auto  FilterContinuousStateAttributes=''  FilterStateMustResolveToSignalObject=off  FilterRTWStateStorageClass=Auto  DifferentiatorICPrevScaledInput=0  DifferentiatorOutMin=[]  DifferentiatorOutMax=[]
  PID Controller1 : simulink/Continuous/PID Controller  Controller=PID  TimeDomain=Continuous-time  SampleTime=-1  IntegratorMethod=Forward Euler  FilterMethod=Forward Euler  Form=Parallel  UseFilter=on  ControllerParametersSource=internal  P=0.1  I=0  D=0  N=100  InitialConditionSource=internal  InitialConditionForIntegrator=0  InitialConditionForFilter=0  ExternalReset=none  LimitOutput=on  UpperSaturationLimit=0.2  LowerSaturationLimit=-0.2  LinearizeAsGain=on  AntiWindupMode=none  Kb=1  TrackingMode=off  Kt=1  PParamMin=[]  PParamMax=[]  IParamMin=[]  IParamMax=[]  DParamMin=[]  DParamMax=[]  NParamMin=[]  NParamMax=[]  KbParamMin=[]  KbParamMax=[]  KtParamMin=[]  KtParamMax=[]  POutMin=[]  POutMax=[]  IOutMin=[]  IOutMax=[]  DOutMin=[]  DOutMax=[]  NOutMin=[]  NOutMax=[]  KbOutMin=[]  KbOutMax=[]  KtOutMin=[]  KtOutMax=[]  IntegratorOutMin=[]  IntegratorOutMax=[]  FilterOutMin=[]  FilterOutMax=[]  SumOutMin=[]  SumOutMax=[]  SumI1OutMin=[]  SumI1OutMax=[]  SumI2OutMin=[]  SumI2OutMax=[]  SumI3OutMin=[]  SumI3OutMax=[]  SumDOutMin=[]  SumDOutMax=[]  SaturationOutMin=[]  SaturationOutMax=[]  IntegratorContinuousStateAttributes=''  IntegratorStateMustResolveToSignalObject=off  IntegratorRTWStateStorageClass=Auto  FilterContinuousStateAttributes=''  FilterStateMustResolveToSignalObject=off  FilterRTWStateStorageClass=Auto  DifferentiatorICPrevScaledInput=0  DifferentiatorOutMin=[]  DifferentiatorOutMax=[]
  PID Controller2 : simulink/Continuous/PID Controller  Controller=PID  TimeDomain=Continuous-time  SampleTime=-1  IntegratorMethod=Forward Euler  FilterMethod=Forward Euler  Form=Parallel  UseFilter=on  ControllerParametersSource=internal  P=0.1  I=0  D=0  N=100  InitialConditionSource=internal  InitialConditionForIntegrator=0  InitialConditionForFilter=0  ExternalReset=none  LimitOutput=on  UpperSaturationLimit=2.5  LowerSaturationLimit=1  LinearizeAsGain=on  AntiWindupMode=none  Kb=1  TrackingMode=off  Kt=1  PParamMin=[]  PParamMax=[]  IParamMin=[]  IParamMax=[]  DParamMin=[]  DParamMax=[]  NParamMin=[]  NParamMax=[]  KbParamMin=[]  KbParamMax=[]  KtParamMin=[]  KtParamMax=[]  POutMin=[]  POutMax=[]  IOutMin=[]  IOutMax=[]  DOutMin=[]  DOutMax=[]  NOutMin=[]  NOutMax=[]  KbOutMin=[]  KbOutMax=[]  KtOutMin=[]  KtOutMax=[]  IntegratorOutMin=[]  IntegratorOutMax=[]  FilterOutMin=[]  FilterOutMax=[]  SumOutMin=[]  SumOutMax=[]  SumI1OutMin=[]  SumI1OutMax=[]  SumI2OutMin=[]  SumI2OutMax=[]  SumI3OutMin=[]  SumI3OutMax=[]  SumDOutMin=[]  SumDOutMax=[]  SaturationOutMin=[]  SaturationOutMax=[]  IntegratorContinuousStateAttributes=''  IntegratorStateMustResolveToSignalObject=off  IntegratorRTWStateStorageClass=Auto  FilterContinuousStateAttributes=''  FilterStateMustResolveToSignalObject=off  FilterRTWStateStorageClass=Auto  DifferentiatorICPrevScaledInput=0  DifferentiatorOutMin=[]  DifferentiatorOutMax=[]
  Product : Product  Multiplication=Matrix(*)
  Rotation Angles to Direction Cosine Matrix : aerolibtransform2/Rotation Angles to Direction Cosine Matrix  rotationOrder=XYZ
  Saturation : Saturate  UpperLimit=0.2  LowerLimit=-0.2
  Scope{,1..3} (4 alike) : Scope
      Scope settings: SaveName=ScopeData5
      Scope1 settings: TimeRange=400  YMin=-150  YMax=200  SaveName=ScopeData6
      Scope2 settings: YMin=5.55112e-17  YMax=1.5  SaveName=ScopeData8
      Scope3 settings: YMin=-35  YMax=40  SaveName=ScopeData9
  Trigonometric Function : Trigonometry  Operator=atan2
  Trigonometric Function1 : Trigonometry
  wrap1 : MATLAB Function  TreatAsAtomicUnit=on
  u : Outport
  w : Outport  Port=2
  wires:
  PID Controller/1 -> PID Controller2/1
  Ye/1 -> Mux1/2
  Xe/1 -> Mux1/1
  Gain2/1 -> Saturation/1, Scope/1
  Gain1/1 -> Trigonometric Function1/1
  Gain/1 -> PID Controller/1
  Demux/2 -> Trigonometric Function/2, Gain/1
  Product/1 -> Demux/1
  Mux1/1 -> Product/2
  Rotation Angles to Direction Cosine Matrix/1 -> Product/1
  Mux/1 -> Rotation Angles to Direction Cosine Matrix/1
  psi/1 -> Mux/3
  Trigonometric Function/1 -> wrap1/1(u), Gain1/1
  Trigonometric Function1/1 -> Gain2/1
  wrap1/1(y) -> Scope2/1
  Demux/1 -> Trigonometric Function/1
  Saturation/1 -> w/1
  PID Controller2/1 -> Scope1/1, u/1

== system PathFollowComp/Range ==
  In1 : Inport
  In2 : Inport  Port=2
  Demux2 : Demux  Outputs=2
  Dot Product2 : DotProduct  InputSameDT=on  OutDataTypeStr=Inherit: Inherit via internal rule
  Dot Product3 : DotProduct  InputSameDT=on  OutDataTypeStr=Inherit: Inherit via internal rule
  Sqrt : Sqrt  SaturateOnIntegerOverflow=on
  Sum4 : Sum  Inputs=+-
  Sum7 : Sum
  Out1 : Outport
  wires:
  Sum7/1 -> Sqrt/1
  Sum4/1 -> Demux2/1
  Dot Product3/1 -> Sum7/2
  Demux2/2 -> Dot Product3/2, Dot Product3/1
  Demux2/1 -> Dot Product2/1, Dot Product2/2
  Dot Product2/1 -> Sum7/1
  Sqrt/1 -> Out1/1
  In1/1 -> Sum4/1
  In2/1 -> Sum4/2

== system PathFollowComp/Range1 ==
  In1 : Inport
  In2 : Inport  Port=2
  Demux2 : Demux  Outputs=2
  Dot Product2 : DotProduct  InputSameDT=on  OutDataTypeStr=Inherit: Inherit via internal rule
  Dot Product3 : DotProduct  InputSameDT=on  OutDataTypeStr=Inherit: Inherit via internal rule
  Sqrt : Sqrt  SaturateOnIntegerOverflow=on
  Sum4 : Sum  Inputs=+-
  Sum7 : Sum
  Out1 : Outport
  wires:
  Sum7/1 -> Sqrt/1
  Sum4/1 -> Demux2/1
  Dot Product3/1 -> Sum7/2
  Demux2/2 -> Dot Product3/2, Dot Product3/1
  Demux2/1 -> Dot Product2/1, Dot Product2/2
  Dot Product2/1 -> Sum7/1
  Sqrt/1 -> Out1/1
  In1/1 -> Sum4/1
  In2/1 -> Sum4/2

== system PathFollowComp/Range2 ==
  In1 : Inport
  In2 : Inport  Port=2
  Demux2 : Demux  Outputs=2
  Dot Product2 : DotProduct  InputSameDT=on  OutDataTypeStr=Inherit: Inherit via internal rule
  Dot Product3 : DotProduct  InputSameDT=on  OutDataTypeStr=Inherit: Inherit via internal rule
  Sqrt : Sqrt  SaturateOnIntegerOverflow=on
  Sum4 : Sum  Inputs=+-
  Sum7 : Sum
  Out1 : Outport
  wires:
  In2/1 -> Sum4/2
  In1/1 -> Sum4/1
  Sqrt/1 -> Out1/1
  Dot Product2/1 -> Sum7/1
  Demux2/1 -> Dot Product2/2, Dot Product2/1
  Demux2/2 -> Dot Product3/1, Dot Product3/2
  Dot Product3/1 -> Sum7/2
  Sum4/1 -> Demux2/1
  Sum7/1 -> Sqrt/1

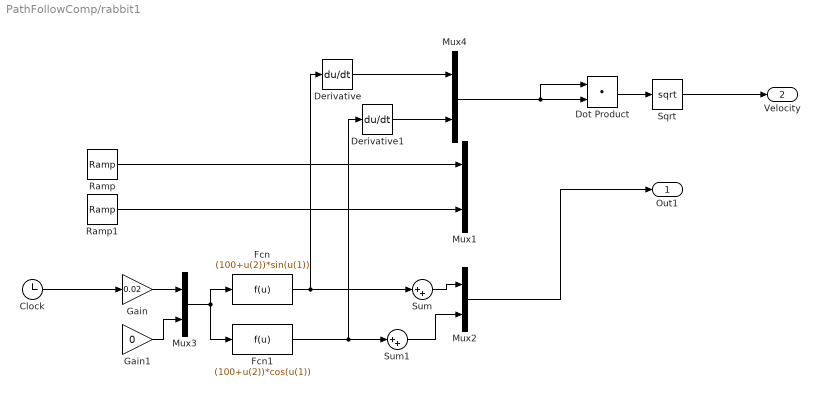
== system PathFollowComp/rabbit1 ==
  Clock : Clock
  Derivative : Derivative
  Derivative1 : Derivative
  Dot Product : DotProduct  InputSameDT=on  OutDataTypeStr=Inherit: Inherit via internal rule
  Fcn : Fcn  Expr=(100+u(2))*sin(u(1))
  Fcn1 : Fcn  Expr=(100+u(2))*cos(u(1))
  Gain : Gain  Gain=0.02
  Gain1 : Gain  Gain=0
  Mux{1..4} (4 alike) : Mux  Inputs=2
  Ramp : simulink/Sources/Ramp  slope=1  start=0  X0=-100
  Ramp1 : simulink/Sources/Ramp  slope=2  start=0  X0=-100
  Sqrt : Sqrt  SaturateOnIntegerOverflow=on
  Sum : Sum  Inputs=|++
  Sum1 : Sum  Inputs=|++
  Out1 : Outport
  Velocity : Outport  Port=2
  wires:
  Ramp/1 -> Mux1/1
  Ramp1/1 -> Mux1/2
  Fcn1/1 -> Derivative1/1, Sum1/1
  Mux3/1 -> Fcn/1, Fcn1/1
  Gain/1 -> Mux3/1
  Gain1/1 -> Mux3/2
  Fcn/1 -> Derivative/1, Sum/1
  Sum/1 -> Mux2/1
  Sum1/1 -> Mux2/2
  Dot Product/1 -> Sqrt/1
  Sqrt/1 -> Velocity/1
  Derivative/1 -> Mux4/1
  Derivative1/1 -> Mux4/2
  Mux4/1 -> Dot Product/1, Dot Product/2
  Mux2/1 -> Out1/1
  Clock/1 -> Gain/1

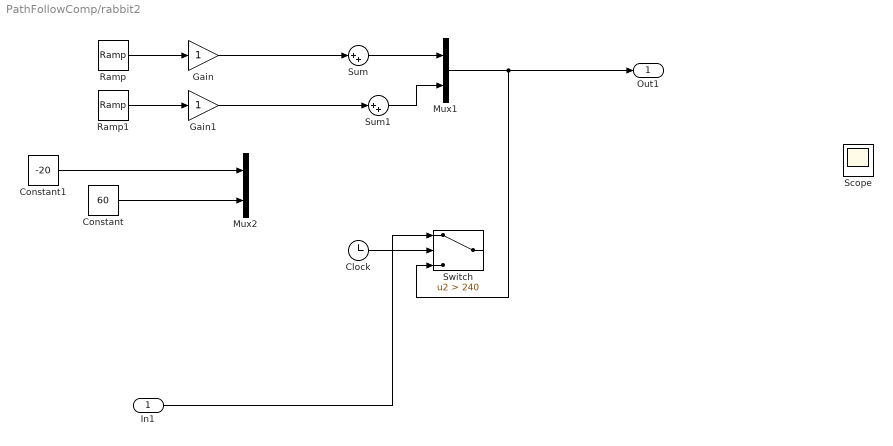
== system PathFollowComp/rabbit2 ==
  In1 : Inport
  Clock : Clock
  Constant : Constant  Value=60
  Constant1 : Constant  Value=-20
  Gain : Gain
  Gain1 : Gain
  Mux1 : Mux  Inputs=2
  Mux2 : Mux  Inputs=2
  Ramp : simulink/Sources/Ramp  slope=-0.5*0  start=0  X0=130
  Ramp1 : simulink/Sources/Ramp  slope=-1*0  start=0  X0=250
  Scope : Scope
      settings: YMin=-25  YMax=300  SaveName=ScopeData4
  Sum : Sum  Inputs=|++
  Sum1 : Sum  Inputs=|++
  Switch : Switch  Criteria=u2 > Threshold  Threshold=240
  Out1 : Outport
  wires:
  Mux1/1 -> Out1/1, Switch/3
  Ramp1/1 -> Gain1/1
  Ramp/1 -> Gain/1
  Gain/1 -> Sum/1
  Gain1/1 -> Sum1/1
  Sum1/1 -> Mux1/2
  Sum/1 -> Mux1/1
  Clock/1 -> Switch/2
  Constant/1 -> Mux2/2
  Constant1/1 -> Mux2/1
  In1/1 -> Switch/1

== system PathFollowComp/Lambda/atan2_unwrap ==
  In1 : Inport
  MATLAB Function1 : MATLAB Function  TreatAsAtomicUnit=on
  Memory : Memory  X0=lambda_0
  Memory1 : Memory
  Out1 : Outport
  wires:
  In1/1 -> Memory/1, MATLAB Function1/1(u)
  Memory/1 -> MATLAB Function1/2(upast)
  MATLAB Function1/1(y) -> Out1/1
  MATLAB Function1/2(bias1) -> Memory1/1
  Memory1/1 -> MATLAB Function1/3(bias)

== system PathFollowComp/Lambda1/atan2_unwrap ==
  In1 : Inport
  MATLAB Function1 : MATLAB Function  TreatAsAtomicUnit=on
  Memory : Memory  X0=lambda_0
  Memory1 : Memory
  Out1 : Outport
  wires:
  In1/1 -> Memory/1, MATLAB Function1/1(u)
  Memory/1 -> MATLAB Function1/2(upast)
  MATLAB Function1/1(y) -> Out1/1
  MATLAB Function1/2(bias1) -> Memory1/1
  Memory1/1 -> MATLAB Function1/3(bias)

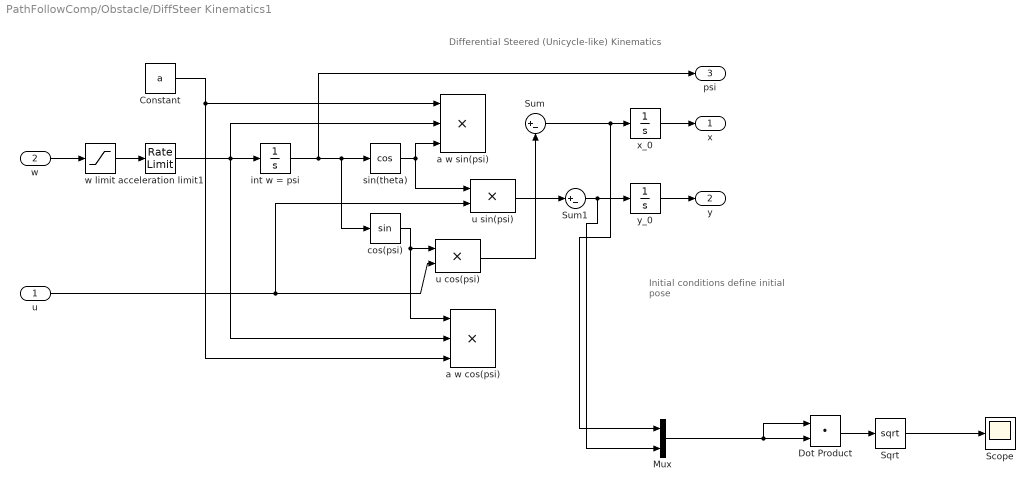
== system PathFollowComp/Obstacle/DiffSteer Kinematics1 ==
  note: Initial conditions define
      | initial pose
  note: Differential Steered (Unicycle-like) Kinematics
  u : Inport
  w : Inport  Port=2
  Constant : Constant  Value=a
  Dot Product : DotProduct  InputSameDT=on  OutDataTypeStr=Inherit: Inherit via internal rule
  Mux : Mux  Inputs=2
  Scope : Scope
      settings: YMin=0  YMax=0.225  SaveName=ScopeData3
  Sqrt : Sqrt  SaturateOnIntegerOverflow=on
  Sum : Sum  Inputs=|+-  SaturateOnIntegerOverflow=on
  Sum1 : Sum  Inputs=|+-  SaturateOnIntegerOverflow=on
  a w cos(psi) : Product  Inputs=3  SaturateOnIntegerOverflow=on  OutDataTypeStr=Inherit: Same as first input
  a w sin(psi) : Product  Inputs=3  SaturateOnIntegerOverflow=on  OutDataTypeStr=Inherit: Same as first input
  acceleration limit1 : RateLimiter  RisingSlewLimit=dwmax  FallingSlewLimit=-dwmax  SampleTimeMode=inherited
  cos(psi) : Trigonometry
  int w = psi : Integrator  InitialCondition=x0(3)
  sin(theta) : Trigonometry  Operator=cos
  u cos(psi) : Product  SaturateOnIntegerOverflow=on  OutDataTypeStr=Inherit: Same as first input
  u sin(psi) : Product  SaturateOnIntegerOverflow=on  OutDataTypeStr=Inherit: Same as first input
  w limit : Saturate  UpperLimit=wmax  LowerLimit=-wmax
  x_0 : Integrator  InitialCondition=x0(1)
  y_0 : Integrator  InitialCondition=x0(2)
  x : Outport
  y : Outport  Port=2
  psi : Outport  Port=3
  wires:
  w limit/1 -> acceleration limit1/1
  w/1 -> w limit/1
  u cos(psi)/1 -> Sum/2
  u sin(psi)/1 -> Sum1/1
  cos(psi)/1 -> u cos(psi)/1, a w cos(psi)/1
  acceleration limit1/1 -> a w sin(psi)/2, int w = psi/1, a w cos(psi)/2
  Constant/1 -> a w sin(psi)/1, a w cos(psi)/3
  x_0/1 -> x/1
  Sum/1 -> Mux/1, x_0/1
  sin(theta)/1 -> a w sin(psi)/3, u sin(psi)/1
  int w = psi/1 -> psi/1, sin(theta)/1, cos(psi)/1
  Sum1/1 -> Mux/2, y_0/1
  y_0/1 -> y/1
  u/1 -> u sin(psi)/2, u cos(psi)/2
  Dot Product/1 -> Sqrt/1
  Sqrt/1 -> Scope/1
  Mux/1 -> Dot Product/1, Dot Product/2

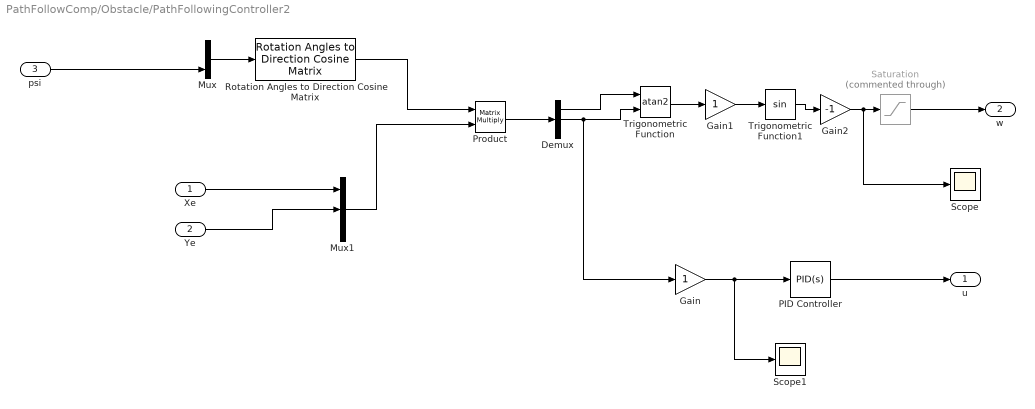
== system PathFollowComp/Obstacle/PathFollowingController2 ==
  Xe : Inport
  Ye : Inport  Port=2
  psi : Inport  Port=3
  Demux : Demux  Outputs=3
  Gain : Gain
  Gain1 : Gain
  Gain2 : Gain  Gain=-1
  Mux : Mux  Inputs=3
  Mux1 : Mux  Inputs=3
  PID Controller : simulink/Continuous/PID Controller  Controller=PID  TimeDomain=Continuous-time  SampleTime=-1  IntegratorMethod=Forward Euler  FilterMethod=Forward Euler  Form=Parallel  UseFilter=on  ControllerParametersSource=internal  P=1.5  I=0  D=0  N=100  InitialConditionSource=internal  InitialConditionForIntegrator=0  InitialConditionForFilter=0  ExternalReset=none  LimitOutput=on  UpperSaturationLimit=1.2  LowerSaturationLimit=0  LinearizeAsGain=on  AntiWindupMode=none  Kb=1  TrackingMode=off  Kt=1  PParamMin=[]  PParamMax=[]  IParamMin=[]  IParamMax=[]  DParamMin=[]  DParamMax=[]  NParamMin=[]  NParamMax=[]  KbParamMin=[]  KbParamMax=[]  KtParamMin=[]  KtParamMax=[]  POutMin=[]  POutMax=[]  IOutMin=[]  IOutMax=[]  DOutMin=[]  DOutMax=[]  NOutMin=[]  NOutMax=[]  KbOutMin=[]  KbOutMax=[]  KtOutMin=[]  KtOutMax=[]  IntegratorOutMin=[]  IntegratorOutMax=[]  FilterOutMin=[]  FilterOutMax=[]  SumOutMin=[]  SumOutMax=[]  SumI1OutMin=[]  SumI1OutMax=[]  SumI2OutMin=[]  SumI2OutMax=[]  SumI3OutMin=[]  SumI3OutMax=[]  SumDOutMin=[]  SumDOutMax=[]  SaturationOutMin=[]  SaturationOutMax=[]  IntegratorContinuousStateAttributes=''  IntegratorStateMustResolveToSignalObject=off  IntegratorRTWStateStorageClass=Auto  FilterContinuousStateAttributes=''  FilterStateMustResolveToSignalObject=off  FilterRTWStateStorageClass=Auto  DifferentiatorICPrevScaledInput=0  DifferentiatorOutMin=[]  DifferentiatorOutMax=[]
  Product : Product  Multiplication=Matrix(*)
  Rotation Angles to Direction Cosine Matrix : aerolibtransform2/Rotation Angles to Direction Cosine Matrix  rotationOrder=XYZ
  Saturation : Saturate  Commented=through
  Scope : Scope
      settings: SaveName=ScopeData5
  Scope1 : Scope
      settings: YMin=8750  YMax=12500  SaveName=ScopeData6
  Trigonometric Function : Trigonometry  Operator=atan2
  Trigonometric Function1 : Trigonometry
  u : Outport
  w : Outport  Port=2
  wires:
  PID Controller/1 -> u/1
  Ye/1 -> Mux1/2
  Xe/1 -> Mux1/1
  Gain2/1 -> Saturation/1, Scope/1
  Gain1/1 -> Trigonometric Function1/1
  Gain/1 -> PID Controller/1, Scope1/1
  Demux/2 -> Trigonometric Function/2, Gain/1
  Product/1 -> Demux/1
  Mux1/1 -> Product/2
  Rotation Angles to Direction Cosine Matrix/1 -> Product/1
  Mux/1 -> Rotation Angles to Direction Cosine Matrix/1
  psi/1 -> Mux/3
  Trigonometric Function/1 -> Gain1/1
  Trigonometric Function1/1 -> Gain2/1
  Demux/1 -> Trigonometric Function/1
  Saturation/1 -> w/1

== matlab function PathFollowComp/Lambda/atan2_unwrap/MATLAB Function1 ==
  data: u input; y output; upast input; bias input; bias1 output
function [y, bias1] = fcn(u,upast,bias)
newbias = 0;
if u-upast > 3*pi/2
    newbias = -4*pi/2;
end
if u-upast < -3*pi/2
   newbias = +4*pi/2;
end
bias1 = bias + newbias;
y = u+bias1;

== matlab function PathFollowComp/Eta/wrap1 ==
  data: u input; y output
function y = fcn(u)
%#codegen

%u2 = mod(u,2*pi);
u2 = u - 2*pi*floor( (u+pi)/(2*pi) ); 
y = u2;

== matlab function PathFollowComp/PathFollowingController1/wrap1 ==
  data: u input; y output
function y = fcn(u)
%#codegen

u2 = mod(u,pi);

y = u2;

== matlab function PathFollowComp/MATLAB Function ==
  data: u1 input; y output; u2 input; range input; flag output; tol input; lambda_dot input; mem input; counter output; eta input; rangethresh input; rhosign input
function [y,flag,counter] = fcn(u1,u2,range,tol, lambda_dot,mem,eta,rangethresh,rhosign)
y=u1;

flag = 0;
if ((range <= rangethresh))
    if ((abs(lambda_dot) < tol) && (eta>0 || rhosign<0) )
        mem = 0;
        y= u2;
        flag = 1;
    end
    if mem > 0
        y= u2;
        flag = 1;
    end
else
    y = u1;
    flag = 0;
end
counter = mem-1;

== matlab function PathFollowComp/PathFollowingController2/wrap1 ==
  data: u input; y output
function y = fcn(u)
%#codegen

u2 = mod(u,pi);

y = u2;

== matlab function PathFollowComp/MATLAB Function1 ==
  data: Xya input; ypast input; u1 input; y output; rabbitvel input; range input; flag output; tol input; lambda_dot input; mem input; counter output; eta input; lambdavec input; y2 output; rangethresh input; rhosign input
function [y,flag,counter,y2] = fcn(Xya,ypast,u1,rabbitvel,range,tol, lambda_dot,mem,eta,lambdavec,rangethresh,rhosign)
y=u1;
returnvec = u1-ypast;
distance = norm(u1-ypast,2);
returnvec = returnvec/(norm(returnvec,2));
y2=u1;
lambdavec = lambdavec/(norm(lambdavec,2));
lambdavecpurp = [0 1; -1 0]*lambdavec;
if ~(eta > -pi/2 || eta <pi/2)
lambdavecpurp = -lambdavecpurp;
end

flag = 0;
if ((range <= rangethresh))
    if ((abs(lambda_dot) < tol) &&((eta > -0.4 || (ypast'*lambdavec>=0) ) && rhosign<0))
        mem = 1500;
         
        y = ypast + lambdavecpurp*rabbitvel*0.01; 
        y2 = ypast + lambdavecpurp*rabbitvel*0.01;
        flag = 1;
    elseif distance > 1
       y = ypast + returnvec*rabbitvel*0.01; 
        y2 = ypast + returnvec*rabbitvel*0.01;
        flag = 2;
    end
else
    y = u1;
    y2 = u1;
    flag = 0;
end
counter = mem -1;
